simulink model "simpleTreeDiff"  (R2024b)
settings: Solver=VariableStepAuto  StartTime=0.0  StopTime=10.0  RelTol=1e-3
settings Model: Creator=neham  LastModifiedBy=neham

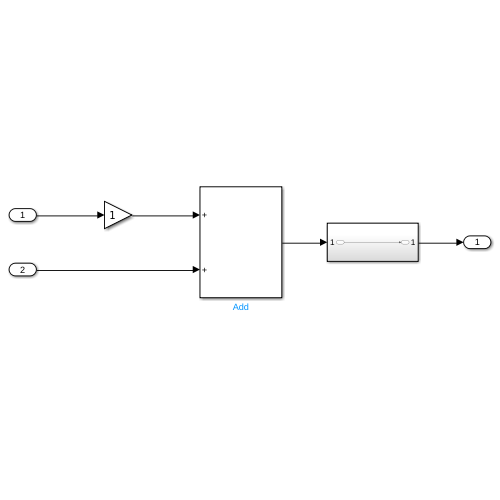
[thumbnail: Simulink's stored preview of the top-level diagram]
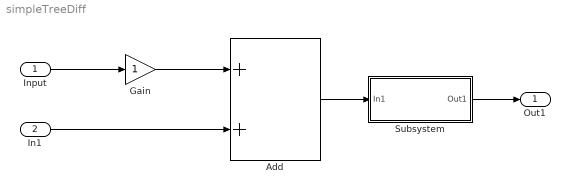
== system simpleTreeDiff ==
  Input : Inport
  In1 : Inport  Port=2
  Add : Sum
  Gain : Gain
  Subsystem : Subsystem
  Out1 : Outport
  wires:
  Input/1 -> Gain/1
  Gain/1 -> Add/1
  In1/1 -> Add/2
  Add/1 -> Subsystem/1(In1)
  Subsystem/1(Out1) -> Out1/1

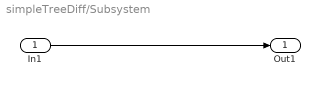
== system simpleTreeDiff/Subsystem ==
  In1 : Inport
  Out1 : Outport
  wires:
  In1/1 -> Out1/1
